simulink model "FlexibleBeam_Test"  (R2021a)
settings: Solver=ode15s  StartTime=0.0  StopTime=10.0  RelTol=1e-3
model workspace (MATLAB code in the model file):
  | % Properties of aluminum
  | alu.rho = 2700; % kg*m^3
  | alu.E   = 70;   % GPa
  | alu.G   = 26;   % GPa
  | 
  | % Properties of fiberglass
  | % https://en.wikipedia.org/wiki/List_of_materials_properties#Mechanical_properties
  | fibG.rho = 1.7;
  | fibG.E = 17.2;
  | fibG.G = 26.0; % not sure of this value
  | 
  | %material = alu;
  | material = fibG;
  | 
  | % Beam length, in m
  | L = 1;
  | 
  | % C-channel cross-sectional geometry
  | % (all dimensions in m)
  | w = 0.1;
  | h = 0.1;
  | t = 0.01;
  | d = max(w,h);
  | w2 = w/2;
  | h2 = h/2;
  | t2 = t/2;
  | h2i = h2 - t2;
  | h2o = h2 + t2;
  | csb = [ -t2 , -h2o ; ...
  |          w  , -h2o ; ...
  |          w  , -h2i ; ...
  |          t2 , -h2i ; ...
  |          t2 ,  h2i ; ...
  |          w  ,  h2i ; ...
  |          w  ,  h2o ; ...
  |         -t2 ,  h2o ];
  | cst = [ -t2 , -h2o ; ...
  |          w  , -h2o ; ...
  |          w  , -h2i ; ...
  |          t2 , -h2i ; ...
  |          t2 , -t2  ; ...
  |          w2 , -t2  ; ...
  |          w2 ,  t2  ; ...
  |          t2 ,  t2  ; ...
  |          t2 ,  h2i ; ...
  |          w  ,  h2i ; ...
  |          w  ,  h2o ; ...
  |         -t2 ,  h2o ; ...
  |         -t2 ,  t2  ; ...
  |         -w2 ,  t2  ; ...
  |         -w2 , -t2  ; ...
  |         -t2 , -t2  ];
  | 
  | % Location of the centroid and shear center
  | % of the C-channel section relative to the
  | % reference frame of the section, in m
  | % (These are obtained from the Derived
  | %  Values section in the dialog for the
  | %  General Flexible Beam block, for the
  | %  specific cross-section defined above.)
  | xc =  0.033;
  | yc =  0;
  | xs = -0.042;
  | ys =  0;
  | 
  | % Properties of the wall
  | wall.dim = [2*d 2*d L/10];
  | wall.rho = alu.rho;
  | wall.clr = [0.4 0.4 0.4];
  | wall.off = -w/4; % offset
  | 
  | % Properties of the beam
  | beam.L   = L;
  | beam.cs  = csb;
  | beam.rho = material.rho;
  | beam.E   = material.E;
  | beam.G   = material.G;
  | beam.bet = 1e-4; % s
  | beam.N   = 2;
  | beam.clr = [0.8 0.8 0.8];
  | 
  | % Properties of rigid tip of the beam
  | tip.t   = t/2;
  | tip.cs  = cst;
  | tip.rho = material.rho;
  | tip.clr = [0.0 1.0 1.0];
  | 
  | % Properties of graphic representations
  | % of cross-sectional centers (reference,
  | % centroid, shear center)
  | grph.dim   = [t t t/2];
  | grph.c.clr = [1.0 0.0 0.0];
  | grph.r.clr = [0.0 0.6 0.0];
  | grph.s.clr = [0.0 0.0 1.0];
  | 
  | % Properties of marker for force/moment
  | % application point
  | mrkr.L   = t/2;
  | mrkr.r   = 0.8*t/2;
  | mrkr.clr = [1.0 1.0 0.0];
undefined symbols (not defined in the file): X, Y, Z
libraries: sm_lib x10, nesl_utility x2
settings Model: Creator=Andy  LastModifiedBy=Andy

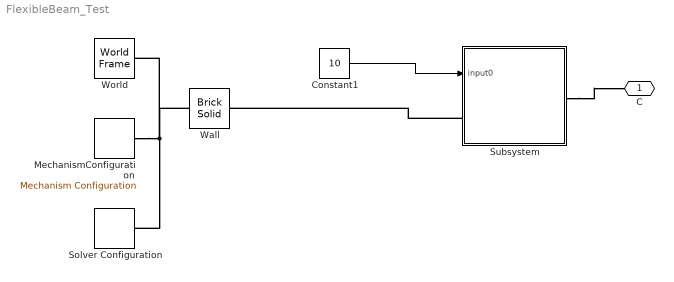
== system FlexibleBeam_Test ==
  Constant1 : Constant  Value=10
  MechanismConfiguration : sm_lib/Utilities/Mechanism Configuration  UniformGravity=Constant  GravityVector=[0 0 -9.80665]*0  GravityVectorUnits=m/s^2  GravityUnits=m/s^2  LinearizationDelta=0.001  JointModeTransitionNonlinearIterations=2
  Solver Configuration : nesl_utility/Solver Configuration  PhysicalDomain=network_engine_domain  SubClassName=solver  LeftPortType=input  RightPortType=generic  Tones=[]  Harmonics=[]  SimulateNoise=off  Profile=off  UseLocalSampling=off  EnableSwitchedLinearOptims=on  FrequencyDomain=off  UseCCode=off  RelTol=0.001  AbsTol=1e-06  MinStep=1e-09  ToWorkspace=off  RevertToSquareIcSolve=off  NumHomotopyIterations=100  PhasorMode=off  PhasorModeNumHarmonics=1  DoDC=off  ResidualTolerance=1e-09  UseLocalSolver=off  LocalSolverChoice=NE_BACKWARD_EULER_ADVANCER  LocalSolverSampleTime=0.001  DoFixedCost=off  MaxNonlinIter=3  MaxModeIter=2  ComputeImpulses=off  ImpulseIterations=2  LinearAlgebra=auto  EquationFormulation=NE_TIME_EF  DelaysMemoryBudget=1024  AutomaticFiltering=on  FilteringTimeConstant=0.001  PartitionStorageMethod=AS_NEEDED  PartitionMemoryBudget=1024  PartitionMethod=ROBUST
      settings: SourceProductBaseCode=PW,SS
  Subsystem : Subsystem
  Wall : sm_lib/Body Elements/Brick Solid  GraphicAmbientColor=[0.15 0.15 0.15 1.0]  BasedOnType=Density  BrickDimensions=wall.dim  BrickDimensionUnits=m  CenterOfMass=[0 0 0]  CenterOfMassUnits=m  GraphicDiffuseColor=wall.clr  Density=wall.rho  DensityUnits=kg/m^3  DoExposeReferenceFrame=on  GraphicEmissiveColor=[0.0 0.0 0.0 1.0]  ExportEntireGeometry=off  SerializedFrames=<Frames><Frame><Id>Frame1</Id><Value><Name>A</Name><Origin><Source>GeometricFeature</Source><FeatureName>+z surface</FeatureName></Origin><PrimaryAxis><DefinedDirection>+Z</DefinedDirection><Source>ReferenceFrame</Source><SourceDirection>+Z</SourceDirection><FeatureName></FeatureName></PrimaryAxis><SecondaryAxis><DefinedDirection>+X</DefinedDirection><Source>ReferenceFrame</Source><SourceDirection>+X</SourceDirection><FeatureName></FeatureName></SecondaryAxis></Value></Frame></Frames>  MarkerShape=Sphere  MarkerSize=10  GraphicType=FromGeometry  InertiaType=CalculateFromGeometry  Mass=1  MassUnits=kg  MomentsOfInertia=[1 1 1]  MomentsOfInertiaUnits=kg*m^2  GraphicOpacity=1.0  ProductsOfInertia=[0 0 0]  ProductsOfInertiaUnits=kg*m^2  GraphicShininess=75  GraphicSpecularColor=[0.5 0.5 0.5 1.0]  GraphicVisPropType=SimpleVisualProperties
  World : sm_lib/Frames and Transforms/World Frame
  C : PMIOPort  Side=Right
  wires:
  Constant1/1 -> Subsystem/1(input0)
  connections:
  MechanismConfiguration/RConn1 -- Wall/RConn1 -- World/RConn1 -- Solver Configuration/RConn1
  Subsystem/LConn1 -- Wall/LConn1
  Subsystem/RConn1 -- C/RConn1

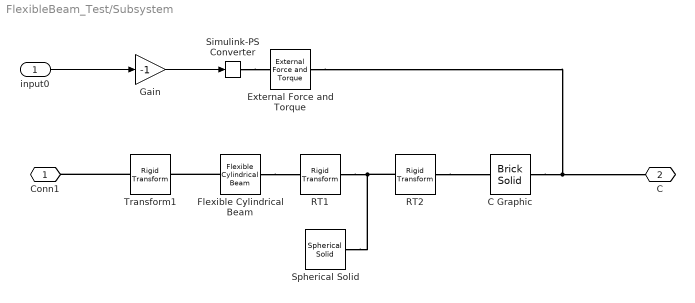
== system FlexibleBeam_Test/Subsystem ==
  input0 : Inport
  C Graphic : sm_lib/Body Elements/Brick Solid  GraphicAmbientColor=[0.15 0.15 0.15 1.0]  BasedOnType=Density  BrickDimensions=grph.dim  BrickDimensionUnits=m  CenterOfMass=[0 0 0]  CenterOfMassUnits=m  GraphicDiffuseColor=grph.c.clr  Density=0  DensityUnits=kg/m^3  DoExposeReferenceFrame=off  GraphicEmissiveColor=[0.0 0.0 0.0 1.0]  ExportEntireGeometry=off  SerializedFrames=<Frames><Frame><Id>Frame1</Id><Value><Name>F</Name><Origin><Source>GeometricFeature</Source><FeatureName>-z surface</FeatureName></Origin><PrimaryAxis><DefinedDirection>+Z</DefinedDirection><Source>ReferenceFrame</Source><SourceDirection>+Z</SourceDirection><FeatureName></FeatureName></PrimaryAxis><SecondaryAxis><DefinedDirection>+X</DefinedDirection><Source>ReferenceFrame</Source><SourceDirection>+X</SourceDirection><FeatureName></FeatureName></SecondaryAxis></Value></Frame><Frame><Id>Frame2</Id><Value><Name>C</Name><Origin><Source>GeometricFeature</Source><FeatureName>+z surface</FeatureName></Origin><PrimaryAxis><DefinedDirection>+Z</DefinedDirection><Source>ReferenceFrame</Source><SourceDirection>+Z</SourceDirection><FeatureName></FeatureName></PrimaryAxis><SecondaryAxis><DefinedDirection>+X</DefinedDirection><Source>ReferenceFrame</Source><SourceDirection>+X</SourceDirection><FeatureName></FeatureName></SecondaryAxis></Value></Frame></Frames>  MarkerShape=Sphere  MarkerSize=10  GraphicType=FromGeometry  InertiaType=CalculateFromGeometry  Mass=1  MassUnits=kg  MomentsOfInertia=[1 1 1]  MomentsOfInertiaUnits=kg*m^2  GraphicOpacity=1.0  ProductsOfInertia=[0 0 0]  ProductsOfInertiaUnits=kg*m^2  GraphicShininess=75  GraphicSpecularColor=[0.5 0.5 0.5 1.0]  GraphicVisPropType=SimpleVisualProperties
  External Force and Torque : sm_lib/Forces and Torques/External Force and Torque  ForceResolutionFrame=AttachedFrame  EnableForceX=off  EnableForceY=off  EnableForceZ=on  EnableForce=off  TorqueResolutionFrame=AttachedFrame  EnableTorqueX=off  EnableTorqueY=off  EnableTorqueZ=off  EnableTorque=off
  Flexible Cylindrical Beam : sm_lib/Body Elements/Flexible Bodies/Beams/Flexible Cylindrical Beam  GraphicAmbientColor=[0.15 0.15 0.15 1.0]  GraphicDiffuseColor=[0.5 0.5 0.5]  SerializedFrames=<Frames/>  DampingType=Proportional  Density=beam.rho  DensityUnits=kg/m^3  DoExposeZmaxFrame=on  DoExposeZminFrame=on  GraphicEmissiveColor=[0.0 0.0 0.0 1.0]  GraphicType=FromGeometry  Length=1  LengthUnits=m  ModuliType=YoungsShear  NumElements=3  GraphicOpacity=1.0  PoissonsRatio=0.33  Radius=0.005  RadiusUnits=m  SectionType=Solid  ShearModulus=beam.G  ShearModulusUnits=GPa  GraphicShininess=75  GraphicSpecularColor=[0.5 0.5 0.5 1.0]  StiffnessType=FromGeometry  Thickness=0.1  ThicknessUnits=m  GraphicVisPropType=SimpleVisualProperties  YoungsModulus=beam.E  YoungsModulusUnits=GPa  ProportionalDampingAlpha=0  ProportionalDampingAlphaUnits=1/s  ProportionalDampingBeta=0.0001  ProportionalDampingBetaUnits=s  UniformModalDampingRatio=0.01
      settings: SourceProductBaseCode=MS
  Gain : Gain  Gain=-1
  RT1 : sm_lib/Frames and Transforms/Rigid Transform  TranslationMethod=StandardAxis  TranslationStandardOffset=0.005/2  TranslationLengthUnit=m  TranslationStandardAxis=+Z  TranslationCartesianOffset=[0 0 0]  TranslationROffset=0  TranslationROffsetUnits=m  TranslationZOffset=0  TranslationZOffsetUnits=m  TranslationThetaOffset=0  TranslationThetaOffsetUnits=deg  RotationMethod=None  RotationAngleUnits=deg  RotationStandardAxis=+Z  RotationAngle=0.0  RotationArbitraryAxis=[0 0 1]  FollAlignAxisA=+X  BaseAlignAxisA=+Y  FollAlignAxisB=+Y  BaseAlignAxisB=+Z  RotationSequenceAxes=FollowerAxes  RotationSequence=XYX  RotationSequenceAngles=[0 0 0]  RotationSequenceAnglesUnits=deg  RotationMatrix=[1 0 0; 0 1 0; 0 0 1]
  RT2 : sm_lib/Frames and Transforms/Rigid Transform  TranslationMethod=StandardAxis  TranslationStandardOffset=0.005/2  TranslationLengthUnit=m  TranslationStandardAxis=+Z  TranslationCartesianOffset=[0 0 0]  TranslationROffset=0  TranslationROffsetUnits=m  TranslationZOffset=0  TranslationZOffsetUnits=m  TranslationThetaOffset=0  TranslationThetaOffsetUnits=deg  RotationMethod=StandardAxis  RotationAngleUnits=deg  RotationStandardAxis=+Y  RotationAngle=0.1  RotationArbitraryAxis=[0 0 1]  FollAlignAxisA=+X  BaseAlignAxisA=+Y  FollAlignAxisB=+Y  BaseAlignAxisB=+Z  RotationSequenceAxes=FollowerAxes  RotationSequence=XYX  RotationSequenceAngles=[0 0 0]  RotationSequenceAnglesUnits=deg  RotationMatrix=[1 0 0; 0 1 0; 0 0 1]
  Simulink-PS Converter : nesl_utility/Simulink-PS Converter  PhysicalDomain=network_engine_domain  SubClassName=ps_input  LeftPortType=input  RightPortType=output  PseudoPeriodic=off  Frequencies=[]  NoiseDistribution=none  NoiseParameters=[]  Unit=1  AffineConversion=off  FilteringAndDerivatives=provide  SimscapeFilterOrder=1  InputFilterTimeConstant=0.001  UdotUserProvided=0
      settings: SourceProductBaseCode=PW,SS
  Spherical Solid : sm_lib/Body Elements/Spherical Solid  GraphicAmbientColor=[0.15 0.15 0.15 1.0]  BasedOnType=Density  CenterOfMass=[0 0 0]  CenterOfMassUnits=m  GraphicDiffuseColor=[0.5 0.5 0.5]  Density=1000  DensityUnits=kg/m^3  DoExposeReferenceFrame=on  GraphicEmissiveColor=[0.0 0.0 0.0 1.0]  ExportEntireGeometry=off  SerializedExposedGeometries=<ExposedGeometries/>  SerializedFrames=<Frames/>  MarkerShape=Sphere  MarkerSize=10  GraphicType=FromGeometry  InertiaType=CalculateFromGeometry  Mass=1  MassUnits=kg  MomentsOfInertia=[1 1 1]  MomentsOfInertiaUnits=kg*m^2  GraphicOpacity=1.0  ProductsOfInertia=[0 0 0]  ProductsOfInertiaUnits=kg*m^2  GraphicShininess=75  GraphicSpecularColor=[0.5 0.5 0.5 1.0]  SphereRadius=0.005  SphereRadiusUnits=m  GraphicVisPropType=SimpleVisualProperties
  Transform1 : sm_lib/Frames and Transforms/Rigid Transform  TranslationMethod=Cartesian  TranslationStandardOffset=0  TranslationLengthUnit=mm  TranslationStandardAxis=+Z  TranslationCartesianOffset=[0 0 0]  TranslationROffset=0  TranslationROffsetUnits=m  TranslationZOffset=0  TranslationZOffsetUnits=m  TranslationThetaOffset=0  TranslationThetaOffsetUnits=deg  RotationMethod=ArbitraryAxis  RotationAngleUnits=deg  RotationStandardAxis=+Z  RotationAngle=90  RotationArbitraryAxis=[0 1 0]  FollAlignAxisA=+X  BaseAlignAxisA=+Y  FollAlignAxisB=+Y  BaseAlignAxisB=+Z  RotationSequenceAxes=FollowerAxes  RotationSequence=XYX  RotationSequenceAngles=[0 0 0]  RotationSequenceAnglesUnits=deg  RotationMatrix=[1 0 0; 0 1 0; 0 0 1]
  Conn1 : PMIOPort  Side=Left
  C : PMIOPort  Port=2  Side=Right
  wires:
  input0/1 -> Gain/1
  Gain/1 -> Simulink-PS Converter/1
  connections:
  Transform1/LConn1 -- Conn1/RConn1
  C Graphic/RConn1 -- C/RConn1 -- External Force and Torque/RConn1
  Flexible Cylindrical Beam/LConn1 -- Transform1/RConn1
  RT1/RConn1 -- RT2/LConn1 -- Spherical Solid/RConn1
  Simulink-PS Converter/RConn1 -- External Force and Torque/LConn1
  RT2/RConn1 -- C Graphic/LConn1
  Flexible Cylindrical Beam/RConn1 -- RT1/LConn1
